simulink model "simulink_elevation_model"  (R2021b)
settings: Solver=FixedStepAuto  StartTime=0.0  StopTime=6  RelTol=1e-3
values from neighbouring files (symbols this model uses):
  fric_gear_motor = 0.0226    [loading_project.m]
  fric_gear_turrent_gun = 100/(185)    (= 0.540540540541)    [loading_project.m]
  ts3 = 10^-3    (= 0.001)    [loading_project.m]
libraries: simulink x4, dspsrcs4 x1
(part 2 of 2)

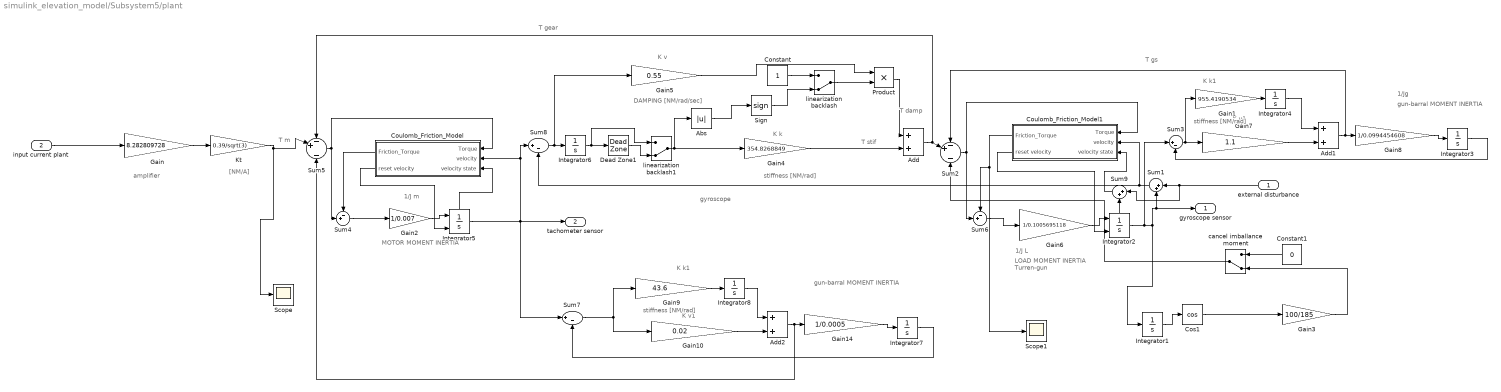
== system simulink_elevation_model/Subsystem5/plant ==
  note: T gs
  note: [NM/A]
  note: K v
  note: amplifier
  note: DAMPING
      | [NM/rad/sec]
  note: K k1
  note: T damp
  note: K v1
  note: stiffness
      | [NM/rad]
  note: 1/J m
  note: MOTOR
      | MOMENT INERTIA
  note: T m
  note: 1/J L
  note: T stif
  note: K k
  note: T gear
  note: LOAD
      | MOMENT INERTIA
      | Turren-gun
  note: stiffness
      | [NM/rad]
  note: gyroscope
  note: gun-barral
      | MOMENT INERTIA
  note: 1/Jg
  note: K v1
  note: K k1
  note: stiffness
      | [NM/rad]
  note: gun-barral
      | MOMENT INERTIA
  external disturbance : Inport
  input current plant : Inport  Port=2
  Abs : Abs
  Add : Sum
  Add1 : Sum
  Add2 : Sum
  Constant : Constant
  Constant1 : Constant  Value=0
  Cos1 : Trigonometry  Operator=cos
  Coulomb_Friction_Model : Subsystem
  Coulomb_Friction_Model1 : Subsystem
  Dead Zone1 : DeadZone  LowerValue=-0.07*10^-3  UpperValue=0.07*10^-3  ZeroCross=off
  Gain : Gain  Gain=8.282809728
  Gain1 : Gain  Gain=955.4190534
  Gain10 : Gain  Gain=0.02
  Gain14 : Gain  Gain=1/0.0005
  Gain2 : Gain  Gain=1/0.007
  Gain3 : Gain  Gain=100/185
  Gain4 : Gain  Gain=354.8268849
  Gain5 : Gain  Gain=0.55
  Gain6 : Gain  Gain=1/0.1005695118
  Gain7 : Gain  Gain=1.1
  Gain8 : Gain  Gain=1/0.0994454608
  Gain9 : Gain  Gain=43.6
  Integrator1 : Integrator  UpperSaturationLimit=pi/2  LowerSaturationLimit=0  WrappedStateUpperValue=pi/2  WrappedStateLowerValue=0
  Integrator2 : Integrator  ExternalReset=rising  ShowStatePort=on  ZeroCross=off
  Integrator{3..4,6..8} (5 alike) : Integrator
  Integrator5 : Integrator  ExternalReset=rising  ShowStatePort=on  ZeroCross=off
  Kt : Gain  Gain=0.39/sqrt(3)
  Product : Product
  Scope : Scope
  Scope1 : Scope
  Sign : Signum
  Sum1 : Sum  Inputs=|++
  Sum2 : Sum  Inputs=-+|-
  Sum3 : Sum  Inputs=|+-
  Sum4 : Sum  Inputs=-+|
  Sum5 : Sum  Inputs=-+|-
  Sum6 : Sum  Inputs=-+|
  Sum7 : Sum  Inputs=|+-
  Sum8 : Sum  Inputs=|+-
  Sum9 : Sum  Inputs=|++
  cancel imballance moment : ManualSwitch  CurrentSetting=0
  linearization backlash : ManualSwitch  CurrentSetting=0
  linearization backlash1 : ManualSwitch  CurrentSetting=0
  gyroscope sensor : Outport
  tachometer sensor : Outport  Port=2
  wires:
  Constant/1 -> linearization backlash/1
  Gain/1 -> Kt/1
  Add/1 -> Sum5/1, Sum2/2
  Integrator4/1 -> Add1/1
  Kt/1 -> Scope/1, Sum5/2
  Gain6/1 -> Integrator2/1
  Gain5/1 -> Product/1
  Gain4/1 -> Add/2
  Sum3/1 -> Gain7/1, Gain1/1
  Sum8/1 -> Gain5/1, Integrator6/1
  Gain2/1 -> Integrator5/1
  Product/1 -> Add/1
  Integrator6/1 -> linearization backlash1/1, Dead Zone1/1
  Abs/1 -> Sign/1
  Gain7/1 -> Add1/2
  linearization backlash/1 -> Product/2
  Integrator3/1 -> Sum3/2
  Sign/1 -> linearization backlash/2
  Gain1/1 -> Integrator4/1
  Sum4/1 -> Gain2/1
  Sum5/1 -> Coulomb_Friction_Model/1(Torque), Sum4/2
  Sum6/1 -> Gain6/1
  Gain8/1 -> Integrator3/1
  Add1/1 -> Gain8/1, Sum2/1
  Integrator2/1 -> Integrator1/1, Sum1/2, gyroscope sensor/1, Sum3/1
  input current plant/1 -> Gain/1
  Sum2/1 -> Sum6/2, Coulomb_Friction_Model1/1(Torque)
  Coulomb_Friction_Model/1(Friction_Torque) -> Sum4/1
  Integrator5/State -> Coulomb_Friction_Model/3(velocity state)
  Coulomb_Friction_Model/2(reset velocity) -> Integrator5/2
  Integrator1/1 -> Cos1/1
  Integrator8/1 -> Add2/1
  Gain9/1 -> Integrator8/1
  Gain10/1 -> Add2/2
  Gain14/1 -> Integrator7/1
  Add2/1 -> Sum5/3, Gain14/1
  Sum7/1 -> Gain10/1, Gain9/1
  Integrator7/1 -> Sum7/2
  Cos1/1 -> Gain3/1
  linearization backlash1/1 -> Abs/1, Gain4/1
  Gain3/1 -> cancel imballance moment/2
  cancel imballance moment/1 -> Sum2/3
  Constant1/1 -> cancel imballance moment/1
  Dead Zone1/1 -> linearization backlash1/2
  Coulomb_Friction_Model1/1(Friction_Torque) -> Sum6/1, Scope1/1
  Coulomb_Friction_Model1/2(reset velocity) -> Integrator2/2
  Sum1/1 -> Coulomb_Friction_Model1/2(velocity), Sum8/2
  Integrator2/State -> Sum9/2
  Sum9/1 -> Coulomb_Friction_Model1/3(velocity state)
  Integrator5/1 -> tachometer sensor/1, Sum7/1, Coulomb_Friction_Model/2(velocity), Sum8/1
  external disturbance/1 -> Sum9/1, Sum1/1

== system simulink_elevation_model/Subsystem6/Subsystem1 ==
  In1 : Inport
  Gain : Gain  Gain=1.6
  Gain1 : Gain  Gain=50
  Integrator : Integrator
  Sum : Sum  Inputs=|++
  Transfer Fcn1 : TransferFcn  Numerator=[1 59.49 9.908*10^4]  Denominator=[1 40 8.72*10^4]
  Transfer Fcn2 : TransferFcn  Numerator=[0.016 1]  Denominator=[0.008 1]
  Transfer Fcn4 : TransferFcn  Numerator=[1 21 1.806*10^4]  Denominator=[1 11.06 9607]
  Transfer Fcn5 : TransferFcn  Numerator=[1 16.78 (2*pi*36)^2]  Denominator=[1 188.3 (2*pi*36)^2]
  Output : Outport
  wires:
  Transfer Fcn5/1 -> Transfer Fcn4/1
  Integrator/1 -> Sum/1
  Gain1/1 -> Integrator/1
  Gain/1 -> Sum/2
  Transfer Fcn4/1 -> Gain/1, Gain1/1
  Sum/1 -> Output/1
  Transfer Fcn1/1 -> Transfer Fcn5/1
  Transfer Fcn2/1 -> Transfer Fcn1/1
  In1/1 -> Transfer Fcn2/1

== system simulink_elevation_model/Subsystem6/Subsystem2 ==
  external distribution : Inport
  Gain : Gain  Gain=1/8.282809728
  Gain1 : Gain  Gain=sqrt(3)/0.39
  Gain2 : Gain  Gain=100/185
  Gain3 : Gain  Gain=-1
  Sign : Signum
  anti friction current : Outport
  wires:
  Gain1/1 -> Gain/1
  Gain3/1 -> Sign/1
  Gain/1 -> anti friction current/1
  Sign/1 -> Gain2/1
  Gain2/1 -> Gain1/1
  external distribution/1 -> Gain3/1

== system simulink_elevation_model/Subsystem6/Subsystem3 ==
  In1 : Inport
  Gain : Gain  Gain=4.5
  Gain1 : Gain
  Gain2 : Gain  Gain=1.8*2*pi
  Integrator : Integrator
  Sum : Sum  Inputs=|++
  Transfer Fcn1 : TransferFcn  Numerator=[1 21 1.806*10^4]  Denominator=[1 25.035 2.102*10^4]
  Transfer Fcn10 : TransferFcn  Numerator=[1 59.495 9.908*10^4]  Denominator=[1 40 8.72*10^4]
  Transfer Fcn7 : TransferFcn  Denominator=[1/(2*pi*6.38)^2 0.55/355 1]
  Transfer Fcn8 : TransferFcn  Numerator=[1 2*0.08*2*35.6*pi (2*pi*35.6)^2]  Denominator=[1 2*0.94*2*35.6*pi (2*pi*35.6)^2]
  Out1 : Outport
  wires:
  Gain/1 -> Gain1/1, Gain2/1
  Sum/1 -> Out1/1
  In1/1 -> Transfer Fcn7/1
  Transfer Fcn8/1 -> Gain/1
  Transfer Fcn7/1 -> Transfer Fcn10/1
  Transfer Fcn10/1 -> Transfer Fcn1/1
  Transfer Fcn1/1 -> Transfer Fcn8/1
  Gain2/1 -> Integrator/1
  Gain1/1 -> Sum/2
  Integrator/1 -> Sum/1

== system simulink_elevation_model/Subsystem6/Subsystem9 ==
  In1 : Inport
  Gain : Gain  Gain=10
  Gain1 : Gain  Gain=26
  Integrator : Integrator
  Sum : Sum  Inputs=|++
  Transfer Fcn4 : TransferFcn  Numerator=[1 2*pi*21.3*2*0.05 (2*pi*21.3)^2]  Denominator=[1 2*pi*21.3*2*0.48 (2*pi*21.3)^2]
  Transfer Fcn5 : TransferFcn  Numerator=[1 16.78 (2*pi*36)^2]  Denominator=[1 188.3 (2*pi*36)^2]
  Output : Outport
  wires:
  Transfer Fcn5/1 -> Transfer Fcn4/1
  In1/1 -> Transfer Fcn5/1
  Integrator/1 -> Sum/1
  Gain1/1 -> Integrator/1
  Gain/1 -> Sum/2
  Transfer Fcn4/1 -> Gain/1, Gain1/1
  Sum/1 -> Output/1

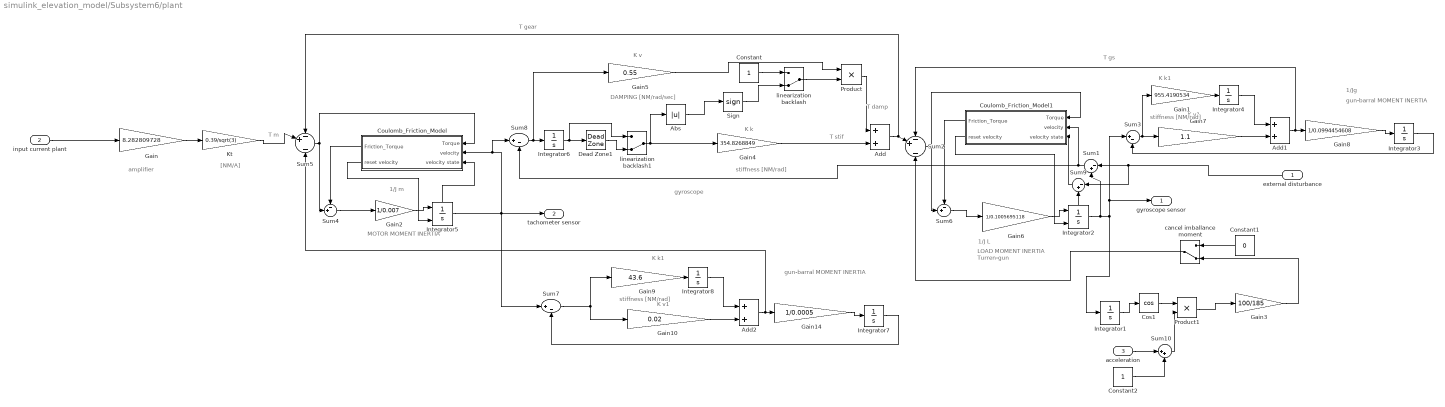
== system simulink_elevation_model/Subsystem6/plant ==
  note: T gs
  note: [NM/A]
  note: K v
  note: amplifier
  note: DAMPING
      | [NM/rad/sec]
  note: K k1
  note: T damp
  note: K v1
  note: stiffness
      | [NM/rad]
  note: 1/J m
  note: MOTOR
      | MOMENT INERTIA
  note: T m
  note: 1/J L
  note: T stif
  note: K k
  note: T gear
  note: LOAD
      | MOMENT INERTIA
      | Turren-gun
  note: stiffness
      | [NM/rad]
  note: gyroscope
  note: gun-barral
      | MOMENT INERTIA
  note: 1/Jg
  note: K v1
  note: K k1
  note: stiffness
      | [NM/rad]
  note: gun-barral
      | MOMENT INERTIA
  external disturbance : Inport
  input current plant : Inport  Port=2
  acceleration : Inport  Port=3
  Abs : Abs
  Add : Sum
  Add1 : Sum
  Add2 : Sum
  Constant : Constant
  Constant1 : Constant  Value=0
  Constant2 : Constant
  Cos1 : Trigonometry  Operator=cos
  Coulomb_Friction_Model : Subsystem
  Coulomb_Friction_Model1 : Subsystem
  Dead Zone1 : DeadZone  LowerValue=-0.07*10^-3  UpperValue=0.07*10^-3  ZeroCross=off
  Gain : Gain  Gain=8.282809728
  Gain1 : Gain  Gain=955.4190534
  Gain10 : Gain  Gain=0.02
  Gain14 : Gain  Gain=1/0.0005
  Gain2 : Gain  Gain=1/0.007
  Gain3 : Gain  Gain=100/185
  Gain4 : Gain  Gain=354.8268849
  Gain5 : Gain  Gain=0.55
  Gain6 : Gain  Gain=1/0.1005695118
  Gain7 : Gain  Gain=1.1
  Gain8 : Gain  Gain=1/0.0994454608
  Gain9 : Gain  Gain=43.6
  Integrator1 : Integrator  UpperSaturationLimit=pi/2  LowerSaturationLimit=0  WrappedStateUpperValue=pi/2  WrappedStateLowerValue=0
  Integrator2 : Integrator  ExternalReset=rising  ShowStatePort=on  ZeroCross=off
  Integrator{3..4,6..8} (5 alike) : Integrator
  Integrator5 : Integrator  ExternalReset=rising  ShowStatePort=on  ZeroCross=off
  Kt : Gain  Gain=0.39/sqrt(3)
  Product : Product
  Product1 : Product
  Sign : Signum
  Sum1 : Sum  Inputs=|-+
  Sum10 : Sum  Inputs=|++
  Sum2 : Sum  Inputs=-+|-
  Sum3 : Sum  Inputs=|+-
  Sum4 : Sum  Inputs=-+|
  Sum5 : Sum  Inputs=-+|-
  Sum6 : Sum  Inputs=-+|
  Sum7 : Sum  Inputs=|+-
  Sum8 : Sum  Inputs=|+-
  Sum9 : Sum  Inputs=|-+
  cancel imballance moment : ManualSwitch  CurrentSetting=0
  linearization backlash : ManualSwitch  CurrentSetting=0
  linearization backlash1 : ManualSwitch  CurrentSetting=0
  gyroscope sensor : Outport
  tachometer sensor : Outport  Port=2
  wires:
  Constant/1 -> linearization backlash/1
  Gain/1 -> Kt/1
  Add/1 -> Sum2/2, Sum5/1
  Integrator4/1 -> Add1/1
  Kt/1 -> Sum5/2
  Gain6/1 -> Integrator2/1
  Gain5/1 -> Product/1
  Gain4/1 -> Add/2
  Sum3/1 -> Gain7/1, Gain1/1
  Sum8/1 -> Gain5/1, Integrator6/1
  Gain2/1 -> Integrator5/1
  Product/1 -> Add/1
  Integrator6/1 -> linearization backlash1/1, Dead Zone1/1
  Abs/1 -> Sign/1
  Gain7/1 -> Add1/2
  linearization backlash/1 -> Product/2
  Integrator3/1 -> Sum3/2
  Sign/1 -> linearization backlash/2
  Gain1/1 -> Integrator4/1
  Sum4/1 -> Gain2/1
  Sum5/1 -> Coulomb_Friction_Model/1(Torque), Sum4/2
  Sum6/1 -> Gain6/1
  Gain8/1 -> Integrator3/1
  Add1/1 -> Gain8/1, Sum2/1
  input current plant/1 -> Gain/1
  Sum2/1 -> Coulomb_Friction_Model1/1(Torque), Sum6/2
  Coulomb_Friction_Model/1(Friction_Torque) -> Sum4/1
  Integrator5/State -> Coulomb_Friction_Model/3(velocity state)
  Coulomb_Friction_Model/2(reset velocity) -> Integrator5/2
  Integrator1/1 -> Cos1/1
  Integrator8/1 -> Add2/1
  Gain9/1 -> Integrator8/1
  Gain10/1 -> Add2/2
  Gain14/1 -> Integrator7/1
  Add2/1 -> Sum5/3, Gain14/1
  Sum7/1 -> Gain10/1, Gain9/1
  Integrator7/1 -> Sum7/2
  linearization backlash1/1 -> Abs/1, Gain4/1
  Gain3/1 -> cancel imballance moment/2
  cancel imballance moment/1 -> Sum2/3
  Constant1/1 -> cancel imballance moment/1
  Dead Zone1/1 -> linearization backlash1/2
  Integrator2/1 -> Integrator1/1, Sum3/1, gyroscope sensor/1, Sum1/2
  Integrator5/1 -> tachometer sensor/1, Sum7/1, Sum8/1, Coulomb_Friction_Model/2(velocity)
  external disturbance/1 -> Sum9/1, Sum1/1
  Sum1/1 -> Coulomb_Friction_Model1/2(velocity), Sum8/2
  Coulomb_Friction_Model1/1(Friction_Torque) -> Sum6/1
  Coulomb_Friction_Model1/2(reset velocity) -> Integrator2/2
  Integrator2/State -> Sum9/2
  Sum9/1 -> Coulomb_Friction_Model1/3(velocity state)
  Cos1/1 -> Product1/1
  Product1/1 -> Gain3/1
  acceleration/1 -> Sum10/1
  Constant2/1 -> Sum10/2
  Sum10/1 -> Product1/2

== system simulink_elevation_model/Subsystem7/Subsystem2 ==
  external distribution : Inport
  Gain : Gain  Gain=1/8.282809728
  Gain1 : Gain  Gain=sqrt(3)/0.39
  Gain2 : Gain  Gain=100/185
  Gain3 : Gain  Gain=-1
  Sign : Signum
  anti friction current : Outport
  wires:
  Gain1/1 -> Gain/1
  external distribution/1 -> Gain3/1
  Gain2/1 -> Gain1/1
  Sign/1 -> Gain2/1
  Gain3/1 -> Sign/1
  Gain/1 -> anti friction current/1

== system simulink_elevation_model/Subsystem7/Subsystem3 ==
  In1 : Inport
  Gain : Gain  Gain=4.5
  Gain1 : Gain
  Gain2 : Gain  Gain=1.8*2*pi
  Integrator : Integrator
  Sum : Sum  Inputs=|++
  Transfer Fcn1 : TransferFcn  Numerator=[1 21 1.806*10^4]  Denominator=[1 25.035 2.102*10^4]
  Transfer Fcn10 : TransferFcn  Numerator=[1 59.495 9.908*10^4]  Denominator=[1 40 8.72*10^4]
  Transfer Fcn7 : TransferFcn  Denominator=[1/(2*pi*6.38)^2 0.55/355 1]
  Transfer Fcn8 : TransferFcn  Numerator=[1 2*0.08*2*35.6*pi (2*pi*35.6)^2]  Denominator=[1 2*0.94*2*35.6*pi (2*pi*35.6)^2]
  Out1 : Outport
  wires:
  Gain/1 -> Gain1/1, Gain2/1
  Sum/1 -> Out1/1
  In1/1 -> Transfer Fcn7/1
  Transfer Fcn8/1 -> Gain/1
  Transfer Fcn7/1 -> Transfer Fcn10/1
  Transfer Fcn10/1 -> Transfer Fcn1/1
  Transfer Fcn1/1 -> Transfer Fcn8/1
  Gain2/1 -> Integrator/1
  Gain1/1 -> Sum/2
  Integrator/1 -> Sum/1

== system simulink_elevation_model/Subsystem7/Subsystem9 ==
  In1 : Inport
  Gain : Gain  Gain=10
  Gain1 : Gain  Gain=26
  Integrator : Integrator
  Sum : Sum  Inputs=|++
  Transfer Fcn4 : TransferFcn  Numerator=[1 2*pi*21.3*2*0.05 (2*pi*21.3)^2]  Denominator=[1 2*pi*21.3*2*0.48 (2*pi*21.3)^2]
  Transfer Fcn5 : TransferFcn  Numerator=[1 16.78 (2*pi*36)^2]  Denominator=[1 188.3 (2*pi*36)^2]
  Output : Outport
  wires:
  Transfer Fcn5/1 -> Transfer Fcn4/1
  In1/1 -> Transfer Fcn5/1
  Integrator/1 -> Sum/1
  Gain1/1 -> Integrator/1
  Gain/1 -> Sum/2
  Transfer Fcn4/1 -> Gain/1, Gain1/1
  Sum/1 -> Output/1

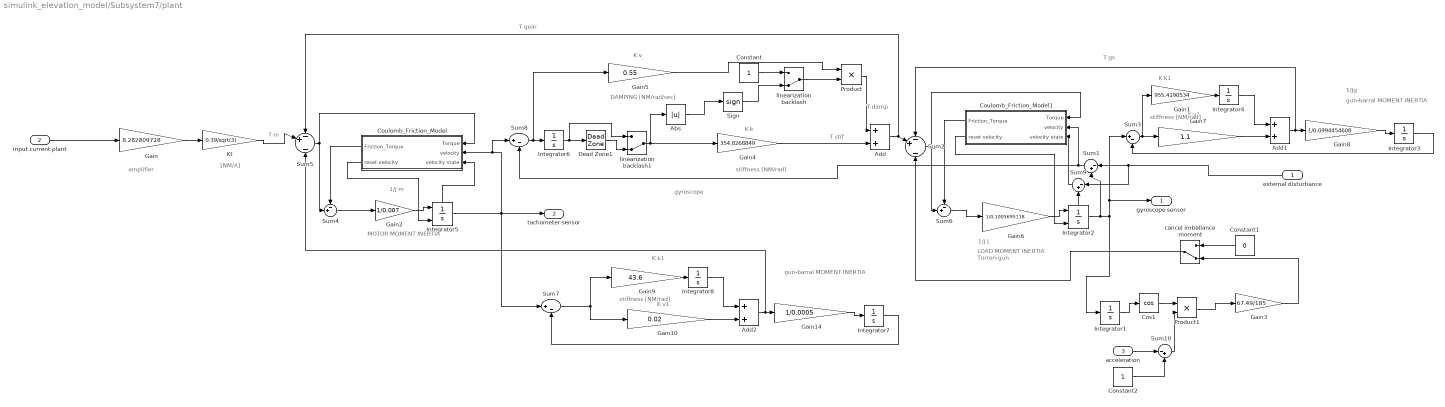
== system simulink_elevation_model/Subsystem7/plant ==
  note: T gs
  note: [NM/A]
  note: K v
  note: amplifier
  note: DAMPING
      | [NM/rad/sec]
  note: K k1
  note: T damp
  note: K v1
  note: stiffness
      | [NM/rad]
  note: 1/J m
  note: MOTOR
      | MOMENT INERTIA
  note: T m
  note: 1/J L
  note: T stif
  note: K k
  note: T gear
  note: LOAD
      | MOMENT INERTIA
      | Turren-gun
  note: stiffness
      | [NM/rad]
  note: gyroscope
  note: gun-barral
      | MOMENT INERTIA
  note: 1/Jg
  note: K v1
  note: K k1
  note: stiffness
      | [NM/rad]
  note: gun-barral
      | MOMENT INERTIA
  external disturbance : Inport
  input current plant : Inport  Port=2
  acceleration : Inport  Port=3
  Abs : Abs
  Add : Sum
  Add1 : Sum
  Add2 : Sum
  Constant : Constant
  Constant1 : Constant  Value=0
  Constant2 : Constant
  Cos1 : Trigonometry  Operator=cos
  Coulomb_Friction_Model : Subsystem
  Coulomb_Friction_Model1 : Subsystem
  Dead Zone1 : DeadZone  LowerValue=-0.07*10^-3  UpperValue=0.07*10^-3  ZeroCross=off
  Gain : Gain  Gain=8.282809728
  Gain1 : Gain  Gain=955.4190534
  Gain10 : Gain  Gain=0.02
  Gain14 : Gain  Gain=1/0.0005
  Gain2 : Gain  Gain=1/0.007
  Gain3 : Gain  Gain=67.49/185
  Gain4 : Gain  Gain=354.8268849
  Gain5 : Gain  Gain=0.55
  Gain6 : Gain  Gain=1/0.1005695118
  Gain7 : Gain  Gain=1.1
  Gain8 : Gain  Gain=1/0.0994454608
  Gain9 : Gain  Gain=43.6
  Integrator1 : Integrator  UpperSaturationLimit=pi/2  LowerSaturationLimit=0  WrappedStateUpperValue=pi/2  WrappedStateLowerValue=0
  Integrator2 : Integrator  ExternalReset=rising  ShowStatePort=on  ZeroCross=off
  Integrator{3..4,6..8} (5 alike) : Integrator
  Integrator5 : Integrator  ExternalReset=rising  ShowStatePort=on  ZeroCross=off
  Kt : Gain  Gain=0.39/sqrt(3)
  Product : Product
  Product1 : Product
  Sign : Signum
  Sum1 : Sum  Inputs=|-+
  Sum10 : Sum  Inputs=|-+
  Sum2 : Sum  Inputs=-+|-
  Sum3 : Sum  Inputs=|+-
  Sum4 : Sum  Inputs=-+|
  Sum5 : Sum  Inputs=-+|-
  Sum6 : Sum  Inputs=-+|
  Sum7 : Sum  Inputs=|+-
  Sum8 : Sum  Inputs=|+-
  Sum9 : Sum  Inputs=|-+
  cancel imballance moment : ManualSwitch  CurrentSetting=0
  linearization backlash : ManualSwitch  CurrentSetting=0
  linearization backlash1 : ManualSwitch  CurrentSetting=0
  gyroscope sensor : Outport
  tachometer sensor : Outport  Port=2
  wires:
  Constant/1 -> linearization backlash/1
  Gain/1 -> Kt/1
  Add/1 -> Sum2/2, Sum5/1
  Integrator4/1 -> Add1/1
  Kt/1 -> Sum5/2
  Gain6/1 -> Integrator2/1
  Gain5/1 -> Product/1
  Gain4/1 -> Add/2
  Sum3/1 -> Gain7/1, Gain1/1
  Sum8/1 -> Gain5/1, Integrator6/1
  Gain2/1 -> Integrator5/1
  Product/1 -> Add/1
  Integrator6/1 -> linearization backlash1/1, Dead Zone1/1
  Abs/1 -> Sign/1
  Gain7/1 -> Add1/2
  linearization backlash/1 -> Product/2
  Integrator3/1 -> Sum3/2
  Sign/1 -> linearization backlash/2
  Gain1/1 -> Integrator4/1
  Sum4/1 -> Gain2/1
  Sum5/1 -> Coulomb_Friction_Model/1(Torque), Sum4/2
  Sum6/1 -> Gain6/1
  Gain8/1 -> Integrator3/1
  Add1/1 -> Gain8/1, Sum2/1
  input current plant/1 -> Gain/1
  Sum2/1 -> Coulomb_Friction_Model1/1(Torque), Sum6/2
  Coulomb_Friction_Model/1(Friction_Torque) -> Sum4/1
  Integrator5/State -> Coulomb_Friction_Model/3(velocity state)
  Coulomb_Friction_Model/2(reset velocity) -> Integrator5/2
  Integrator1/1 -> Cos1/1
  Integrator8/1 -> Add2/1
  Gain9/1 -> Integrator8/1
  Gain10/1 -> Add2/2
  Gain14/1 -> Integrator7/1
  Add2/1 -> Sum5/3, Gain14/1
  Sum7/1 -> Gain10/1, Gain9/1
  Integrator7/1 -> Sum7/2
  linearization backlash1/1 -> Abs/1, Gain4/1
  Gain3/1 -> cancel imballance moment/2
  cancel imballance moment/1 -> Sum2/3
  Constant1/1 -> cancel imballance moment/1
  Dead Zone1/1 -> linearization backlash1/2
  Integrator2/1 -> Integrator1/1, Sum3/1, gyroscope sensor/1, Sum1/2
  Integrator5/1 -> tachometer sensor/1, Sum7/1, Sum8/1, Coulomb_Friction_Model/2(velocity)
  external disturbance/1 -> Sum9/1, Sum1/1
  Sum1/1 -> Coulomb_Friction_Model1/2(velocity), Sum8/2
  Coulomb_Friction_Model1/1(Friction_Torque) -> Sum6/1
  Coulomb_Friction_Model1/2(reset velocity) -> Integrator2/2
  Integrator2/State -> Sum9/2
  Sum9/1 -> Coulomb_Friction_Model1/3(velocity state)
  Cos1/1 -> Product1/1
  Product1/1 -> Gain3/1
  acceleration/1 -> Sum10/1
  Constant2/1 -> Sum10/2
  Sum10/1 -> Product1/2

== system simulink_elevation_model/linear_plant/Coulomb_Friction_Model ==
  Torque : Inport
  velocity : Inport  Port=2
  velocity state : Inport  Port=3
  Abs2 : Abs  ZeroCross=off
  Gain : Gain  Gain=0
  Gain1 : Gain  Gain=0
  Hit Crossing : HitCross  ZeroCross=off
  MinMax : MinMax  Inputs=2
  Product1 : Product  RndMeth=Zero
  Product2 : Product  RndMeth=Zero
  Sign1 : Signum  ZeroCross=off
  Sign2 : Signum  ZeroCross=off
  Slip_T_friction : Constant  Value=fric_gear_motor
  Stick_T_friction : Constant  Value=fric_gear_motor
  Sw6 : Switch  Threshold=0.5  ZeroCross=off  SaturateOnIntegerOverflow=on  InputSameDT=on
  Friction_Torque : Outport
  reset velocity : Outport  Port=2
  wires:
  Torque/1 -> Sign1/1, Abs2/1
  Sw6/1 -> Friction_Torque/1
  Hit Crossing/1 -> reset velocity/1, Sw6/2
  Abs2/1 -> MinMax/2
  MinMax/1 -> Product2/1
  Product2/1 -> Sw6/1
  Product1/1 -> Sw6/3
  Sign2/1 -> Product1/2
  velocity/1 -> Sign2/1
  Sign1/1 -> Product2/2
  velocity state/1 -> Hit Crossing/1
  Stick_T_friction/1 -> Gain/1
  Gain/1 -> MinMax/1
  Slip_T_friction/1 -> Gain1/1
  Gain1/1 -> Product1/1

== system simulink_elevation_model/linear_plant/Coulomb_Friction_Model1 ==
  Torque : Inport
  velocity : Inport  Port=2
  velocity state : Inport  Port=3
  Abs2 : Abs  ZeroCross=off
  Gain : Gain  Gain=0
  Gain1 : Gain  Gain=0
  Hit Crossing : HitCross  ZeroCross=off
  MinMax : MinMax  Inputs=2
  Product1 : Product  RndMeth=Zero
  Product2 : Product  RndMeth=Zero
  Sign1 : Signum  ZeroCross=off
  Sign2 : Signum  ZeroCross=off
  Slip_T_friction : Constant  Value=fric_gear_turrent_gun  SampleTime=0
  Stick_T_friction : Constant  Value=fric_gear_turrent_gun  SampleTime=0
  Sw6 : Switch  Threshold=0.5  ZeroCross=off  SaturateOnIntegerOverflow=on  InputSameDT=on
  Friction_Torque : Outport
  reset velocity : Outport  Port=2
  wires:
  Torque/1 -> Sign2/1, Abs2/1
  Sw6/1 -> Friction_Torque/1
  Hit Crossing/1 -> reset velocity/1, Sw6/2
  Abs2/1 -> MinMax/2
  MinMax/1 -> Product2/1
  Product2/1 -> Sw6/1
  Product1/1 -> Sw6/3
  velocity/1 -> Sign1/1
  Sign1/1 -> Product1/2
  Sign2/1 -> Product2/2
  velocity state/1 -> Hit Crossing/1
  Gain/1 -> MinMax/1
  Stick_T_friction/1 -> Gain/1
  Slip_T_friction/1 -> Gain1/1
  Gain1/1 -> Product1/1

== system simulink_elevation_model/Subsystem2/plant/Coulomb_Friction_Model ==
  Torque : Inport
  velocity : Inport  Port=2
  velocity state : Inport  Port=3
  Abs2 : Abs  ZeroCross=off
  Gain : Gain  Gain=0
  Gain2 : Gain  Gain=0
  Hit Crossing : HitCross  ZeroCross=off
  MinMax : MinMax  Inputs=2
  Product1 : Product  RndMeth=Zero
  Product2 : Product  RndMeth=Zero
  Sign1 : Signum  ZeroCross=off
  Sign2 : Signum  ZeroCross=off
  Slip_T_friction : Constant  Value=fric_gear_motor
  Stick_T_friction : Constant  Value=fric_gear_motor
  Sw6 : Switch  Threshold=0.5  ZeroCross=off  SaturateOnIntegerOverflow=on  InputSameDT=on
  Friction_Torque : Outport
  reset velocity : Outport  Port=2
  wires:
  Torque/1 -> Sign1/1, Abs2/1
  Sw6/1 -> Friction_Torque/1
  Hit Crossing/1 -> reset velocity/1, Sw6/2
  Abs2/1 -> MinMax/2
  MinMax/1 -> Product2/1
  Product2/1 -> Sw6/1
  Product1/1 -> Sw6/3
  Stick_T_friction/1 -> Gain2/1
  Gain2/1 -> MinMax/1
  Sign2/1 -> Product1/2
  velocity/1 -> Sign2/1
  Sign1/1 -> Product2/2
  velocity state/1 -> Hit Crossing/1
  Slip_T_friction/1 -> Gain/1
  Gain/1 -> Product1/1

== system simulink_elevation_model/Subsystem2/plant/Coulomb_Friction_Model1 ==
  Torque : Inport
  velocity : Inport  Port=2
  velocity state : Inport  Port=3
  Abs2 : Abs  ZeroCross=off
  Gain : Gain  Gain=0
  Gain2 : Gain  Gain=0
  Hit Crossing : HitCross  ZeroCross=off
  MinMax : MinMax  Inputs=2
  Product1 : Product  RndMeth=Zero
  Product2 : Product  RndMeth=Zero
  Sign1 : Signum  ZeroCross=off
  Sign2 : Signum  ZeroCross=off
  Slip_T_friction : Constant  Value=fric_gear_turrent_gun  SampleTime=0
  Stick_T_friction : Constant  Value=fric_gear_turrent_gun  SampleTime=0
  Sw6 : Switch  Threshold=0.5  ZeroCross=off  SaturateOnIntegerOverflow=on  InputSameDT=on
  Friction_Torque : Outport
  reset velocity : Outport  Port=2
  wires:
  Torque/1 -> Sign2/1, Abs2/1
  Sw6/1 -> Friction_Torque/1
  Hit Crossing/1 -> reset velocity/1, Sw6/2
  Abs2/1 -> MinMax/2
  MinMax/1 -> Product2/1
  Product2/1 -> Sw6/1
  Product1/1 -> Sw6/3
  Stick_T_friction/1 -> Gain2/1
  Gain2/1 -> MinMax/1
  velocity/1 -> Sign1/1
  Sign1/1 -> Product1/2
  Sign2/1 -> Product2/2
  velocity state/1 -> Hit Crossing/1
  Slip_T_friction/1 -> Gain/1
  Gain/1 -> Product1/1

== system simulink_elevation_model/Subsystem3/plant/Coulomb_Friction_Model ==
  Torque : Inport
  velocity : Inport  Port=2
  velocity state : Inport  Port=3
  Abs2 : Abs  ZeroCross=off
  Gain : Gain
  Gain2 : Gain  Gain=1.1
  Hit Crossing : HitCross  ZeroCross=off
  MinMax : MinMax  Inputs=2
  Product1 : Product  RndMeth=Zero
  Product2 : Product  RndMeth=Zero
  Sign1 : Signum  ZeroCross=off
  Sign2 : Signum  ZeroCross=off
  Slip_T_friction : Constant  Value=fric_gear_motor
  Stick_T_friction : Constant  Value=fric_gear_motor
  Sw6 : Switch  Threshold=0.5  ZeroCross=off  SaturateOnIntegerOverflow=on  InputSameDT=on
  Friction_Torque : Outport
  reset velocity : Outport  Port=2
  wires:
  Torque/1 -> Sign1/1, Abs2/1
  Sw6/1 -> Friction_Torque/1
  Hit Crossing/1 -> reset velocity/1, Sw6/2
  Abs2/1 -> MinMax/2
  MinMax/1 -> Product2/1
  Product2/1 -> Sw6/1
  Product1/1 -> Sw6/3
  Stick_T_friction/1 -> Gain2/1
  Gain2/1 -> MinMax/1
  Sign2/1 -> Product1/2
  velocity/1 -> Sign2/1
  Sign1/1 -> Product2/2
  velocity state/1 -> Hit Crossing/1
  Slip_T_friction/1 -> Gain/1
  Gain/1 -> Product1/1

== system simulink_elevation_model/Subsystem3/plant/Coulomb_Friction_Model1 ==
  Torque : Inport
  velocity : Inport  Port=2
  velocity state : Inport  Port=3
  Abs2 : Abs  ZeroCross=off
  Gain : Gain
  Gain2 : Gain  Gain=1.1
  Hit Crossing : HitCross  ZeroCross=off
  MinMax : MinMax  Inputs=2
  Product1 : Product  RndMeth=Zero
  Product2 : Product  RndMeth=Zero
  Sign1 : Signum  ZeroCross=off
  Sign2 : Signum  ZeroCross=off
  Slip_T_friction : Constant  Value=fric_gear_turrent_gun  SampleTime=0
  Stick_T_friction : Constant  Value=fric_gear_turrent_gun  SampleTime=0
  Sw6 : Switch  Threshold=0.5  ZeroCross=off  SaturateOnIntegerOverflow=on  InputSameDT=on
  Friction_Torque : Outport
  reset velocity : Outport  Port=2
  wires:
  Torque/1 -> Sign2/1, Abs2/1
  Sw6/1 -> Friction_Torque/1
  Hit Crossing/1 -> reset velocity/1, Sw6/2
  Abs2/1 -> MinMax/2
  MinMax/1 -> Product2/1
  Product2/1 -> Sw6/1
  Product1/1 -> Sw6/3
  Stick_T_friction/1 -> Gain2/1
  Gain2/1 -> MinMax/1
  velocity/1 -> Sign1/1
  Sign1/1 -> Product1/2
  Sign2/1 -> Product2/2
  velocity state/1 -> Hit Crossing/1
  Slip_T_friction/1 -> Gain/1
  Gain/1 -> Product1/1

== system simulink_elevation_model/Subsystem4/plant/Coulomb_Friction_Model ==
  Torque : Inport
  velocity : Inport  Port=2
  velocity state : Inport  Port=3
  Abs2 : Abs  ZeroCross=off
  Gain2 : Gain  Gain=1.1
  Hit Crossing : HitCross  ZeroCross=off
  MinMax : MinMax  Inputs=2
  Product1 : Product  RndMeth=Zero
  Product2 : Product  RndMeth=Zero
  Sign1 : Signum  ZeroCross=off
  Sign2 : Signum  ZeroCross=off
  Slip_T_friction : Constant  Value=fric_gear_motor
  Stick_T_friction : Constant  Value=fric_gear_motor
  Sw6 : Switch  Threshold=0.5  ZeroCross=off  SaturateOnIntegerOverflow=on  InputSameDT=on
  Friction_Torque : Outport
  reset velocity : Outport  Port=2
  wires:
  Torque/1 -> Sign1/1, Abs2/1
  Sw6/1 -> Friction_Torque/1
  Hit Crossing/1 -> reset velocity/1, Sw6/2
  Abs2/1 -> MinMax/2
  MinMax/1 -> Product2/1
  Slip_T_friction/1 -> Product1/1
  Product2/1 -> Sw6/1
  Product1/1 -> Sw6/3
  Stick_T_friction/1 -> Gain2/1
  Gain2/1 -> MinMax/1
  Sign2/1 -> Product1/2
  velocity/1 -> Sign2/1
  Sign1/1 -> Product2/2
  velocity state/1 -> Hit Crossing/1

== system simulink_elevation_model/Subsystem4/plant/Coulomb_Friction_Model1 ==
  Torque : Inport
  velocity : Inport  Port=2
  velocity state : Inport  Port=3
  Abs2 : Abs  ZeroCross=off
  Gain2 : Gain  Gain=1.1
  Hit Crossing : HitCross  ZeroCross=off
  MinMax : MinMax  Inputs=2
  Product1 : Product  RndMeth=Zero
  Product2 : Product  RndMeth=Zero
  Sign1 : Signum  ZeroCross=off
  Sign2 : Signum  ZeroCross=off
  Slip_T_friction : Constant  Value=fric_gear_turrent_gun  SampleTime=0
  Stick_T_friction : Constant  Value=fric_gear_turrent_gun  SampleTime=0
  Sw6 : Switch  Threshold=0.5  ZeroCross=off  SaturateOnIntegerOverflow=on  InputSameDT=on
  Friction_Torque : Outport
  reset velocity : Outport  Port=2
  wires:
  Torque/1 -> Sign2/1, Abs2/1
  Sw6/1 -> Friction_Torque/1
  Hit Crossing/1 -> reset velocity/1, Sw6/2
  Abs2/1 -> MinMax/2
  MinMax/1 -> Product2/1
  Slip_T_friction/1 -> Product1/1
  Product2/1 -> Sw6/1
  Product1/1 -> Sw6/3
  Stick_T_friction/1 -> Gain2/1
  Gain2/1 -> MinMax/1
  velocity/1 -> Sign1/1
  Sign1/1 -> Product1/2
  Sign2/1 -> Product2/2
  velocity state/1 -> Hit Crossing/1

== system simulink_elevation_model/Subsystem5/plant/Coulomb_Friction_Model ==
  Torque : Inport
  velocity : Inport  Port=2
  velocity state : Inport  Port=3
  Abs2 : Abs  ZeroCross=off
  Gain : Gain  Gain=1.1
  Gain1 : Gain
  Hit Crossing : HitCross  ZeroCross=off
  MinMax : MinMax  Inputs=2
  Product1 : Product  RndMeth=Zero
  Product2 : Product  RndMeth=Zero
  Sign1 : Signum  ZeroCross=off
  Sign2 : Signum  ZeroCross=off
  Slip_T_friction : Constant  Value=fric_gear_motor
  Stick_T_friction : Constant  Value=fric_gear_motor
  Sw6 : Switch  Threshold=0.5  ZeroCross=off  SaturateOnIntegerOverflow=on  InputSameDT=on
  Friction_Torque : Outport
  reset velocity : Outport  Port=2
  wires:
  Torque/1 -> Sign1/1, Abs2/1
  Sw6/1 -> Friction_Torque/1
  Hit Crossing/1 -> reset velocity/1, Sw6/2
  Abs2/1 -> MinMax/2
  MinMax/1 -> Product2/1
  Product2/1 -> Sw6/1
  Product1/1 -> Sw6/3
  Sign2/1 -> Product1/2
  velocity/1 -> Sign2/1
  Sign1/1 -> Product2/2
  velocity state/1 -> Hit Crossing/1
  Stick_T_friction/1 -> Gain/1
  Gain/1 -> MinMax/1
  Slip_T_friction/1 -> Gain1/1
  Gain1/1 -> Product1/1

== system simulink_elevation_model/Subsystem5/plant/Coulomb_Friction_Model1 ==
  Torque : Inport
  velocity : Inport  Port=2
  velocity state : Inport  Port=3
  Abs2 : Abs  ZeroCross=off
  Gain : Gain  Gain=1.1
  Gain1 : Gain
  Hit Crossing : HitCross  ZeroCross=off
  MinMax : MinMax  Inputs=2
  Product1 : Product  RndMeth=Zero
  Product2 : Product  RndMeth=Zero
  Sign1 : Signum  ZeroCross=off
  Sign2 : Signum  ZeroCross=off
  Slip_T_friction : Constant  Value=fric_gear_turrent_gun  SampleTime=0
  Stick_T_friction : Constant  Value=fric_gear_turrent_gun  SampleTime=0
  Sw6 : Switch  Threshold=0.5  ZeroCross=off  SaturateOnIntegerOverflow=on  InputSameDT=on
  Friction_Torque : Outport
  reset velocity : Outport  Port=2
  wires:
  Torque/1 -> Sign2/1, Abs2/1
  Sw6/1 -> Friction_Torque/1
  Hit Crossing/1 -> reset velocity/1, Sw6/2
  Abs2/1 -> MinMax/2
  MinMax/1 -> Product2/1
  Product2/1 -> Sw6/1
  Product1/1 -> Sw6/3
  velocity/1 -> Sign1/1
  Sign1/1 -> Product1/2
  Sign2/1 -> Product2/2
  velocity state/1 -> Hit Crossing/1
  Gain/1 -> MinMax/1
  Stick_T_friction/1 -> Gain/1
  Slip_T_friction/1 -> Gain1/1
  Gain1/1 -> Product1/1

== system simulink_elevation_model/Subsystem6/plant/Coulomb_Friction_Model ==
  Torque : Inport
  velocity : Inport  Port=2
  velocity state : Inport  Port=3
  Abs2 : Abs  ZeroCross=off
  Gain2 : Gain  Gain=1.1
  Hit Crossing : HitCross  ZeroCross=off
  MinMax : MinMax  Inputs=2
  Product1 : Product  RndMeth=Zero
  Product2 : Product  RndMeth=Zero
  Sign1 : Signum  ZeroCross=off
  Sign2 : Signum  ZeroCross=off
  Slip_T_friction : Constant  Value=fric_gear_motor
  Stick_T_friction : Constant  Value=fric_gear_motor
  Sw6 : Switch  Threshold=0.5  ZeroCross=off  SaturateOnIntegerOverflow=on  InputSameDT=on
  Friction_Torque : Outport
  reset velocity : Outport  Port=2
  wires:
  Torque/1 -> Sign1/1, Abs2/1
  Sw6/1 -> Friction_Torque/1
  Hit Crossing/1 -> reset velocity/1, Sw6/2
  Abs2/1 -> MinMax/2
  MinMax/1 -> Product2/1
  Slip_T_friction/1 -> Product1/1
  Product2/1 -> Sw6/1
  Product1/1 -> Sw6/3
  Stick_T_friction/1 -> Gain2/1
  Gain2/1 -> MinMax/1
  Sign2/1 -> Product1/2
  velocity/1 -> Sign2/1
  Sign1/1 -> Product2/2
  velocity state/1 -> Hit Crossing/1

== system simulink_elevation_model/Subsystem6/plant/Coulomb_Friction_Model1 ==
  Torque : Inport
  velocity : Inport  Port=2
  velocity state : Inport  Port=3
  Abs2 : Abs  ZeroCross=off
  Gain2 : Gain  Gain=1.1
  Hit Crossing : HitCross  ZeroCross=off
  MinMax : MinMax  Inputs=2
  Product1 : Product  RndMeth=Zero
  Product2 : Product  RndMeth=Zero
  Sign1 : Signum  ZeroCross=off
  Sign2 : Signum  ZeroCross=off
  Slip_T_friction : Constant  Value=fric_gear_turrent_gun  SampleTime=0
  Stick_T_friction : Constant  Value=fric_gear_turrent_gun  SampleTime=0
  Sw6 : Switch  Threshold=0.5  ZeroCross=off  SaturateOnIntegerOverflow=on  InputSameDT=on
  Friction_Torque : Outport
  reset velocity : Outport  Port=2
  wires:
  Torque/1 -> Sign2/1, Abs2/1
  Sw6/1 -> Friction_Torque/1
  Hit Crossing/1 -> reset velocity/1, Sw6/2
  Abs2/1 -> MinMax/2
  MinMax/1 -> Product2/1
  Slip_T_friction/1 -> Product1/1
  Product2/1 -> Sw6/1
  Product1/1 -> Sw6/3
  Stick_T_friction/1 -> Gain2/1
  Gain2/1 -> MinMax/1
  velocity/1 -> Sign1/1
  Sign1/1 -> Product1/2
  Sign2/1 -> Product2/2
  velocity state/1 -> Hit Crossing/1

== system simulink_elevation_model/Subsystem7/plant/Coulomb_Friction_Model ==
  Torque : Inport
  velocity : Inport  Port=2
  velocity state : Inport  Port=3
  Abs2 : Abs  ZeroCross=off
  Gain2 : Gain  Gain=1.1
  Hit Crossing : HitCross  ZeroCross=off
  MinMax : MinMax  Inputs=2
  Product1 : Product  RndMeth=Zero
  Product2 : Product  RndMeth=Zero
  Sign1 : Signum  ZeroCross=off
  Sign2 : Signum  ZeroCross=off
  Slip_T_friction : Constant  Value=fric_gear_motor
  Stick_T_friction : Constant  Value=fric_gear_motor
  Sw6 : Switch  Threshold=0.5  ZeroCross=off  SaturateOnIntegerOverflow=on  InputSameDT=on
  Friction_Torque : Outport
  reset velocity : Outport  Port=2
  wires:
  Torque/1 -> Sign1/1, Abs2/1
  Sw6/1 -> Friction_Torque/1
  Hit Crossing/1 -> reset velocity/1, Sw6/2
  Abs2/1 -> MinMax/2
  MinMax/1 -> Product2/1
  Slip_T_friction/1 -> Product1/1
  Product2/1 -> Sw6/1
  Product1/1 -> Sw6/3
  Stick_T_friction/1 -> Gain2/1
  Gain2/1 -> MinMax/1
  Sign2/1 -> Product1/2
  velocity/1 -> Sign2/1
  Sign1/1 -> Product2/2
  velocity state/1 -> Hit Crossing/1

== system simulink_elevation_model/Subsystem7/plant/Coulomb_Friction_Model1 ==
  Torque : Inport
  velocity : Inport  Port=2
  velocity state : Inport  Port=3
  Abs2 : Abs  ZeroCross=off
  Gain2 : Gain  Gain=1.1
  Hit Crossing : HitCross  ZeroCross=off
  MinMax : MinMax  Inputs=2
  Product1 : Product  RndMeth=Zero
  Product2 : Product  RndMeth=Zero
  Sign1 : Signum  ZeroCross=off
  Sign2 : Signum  ZeroCross=off
  Slip_T_friction : Constant  Value=fric_gear_turrent_gun  SampleTime=0
  Stick_T_friction : Constant  Value=fric_gear_turrent_gun  SampleTime=0
  Sw6 : Switch  Threshold=0.5  ZeroCross=off  SaturateOnIntegerOverflow=on  InputSameDT=on
  Friction_Torque : Outport
  reset velocity : Outport  Port=2
  wires:
  Torque/1 -> Sign2/1, Abs2/1
  Sw6/1 -> Friction_Torque/1
  Hit Crossing/1 -> reset velocity/1, Sw6/2
  Abs2/1 -> MinMax/2
  MinMax/1 -> Product2/1
  Slip_T_friction/1 -> Product1/1
  Product2/1 -> Sw6/1
  Product1/1 -> Sw6/3
  Stick_T_friction/1 -> Gain2/1
  Gain2/1 -> MinMax/1
  velocity/1 -> Sign1/1
  Sign1/1 -> Product1/2
  Sign2/1 -> Product2/2
  velocity state/1 -> Hit Crossing/1
